simulink subsystem "Heater_Control"  (R2024b)
settings: Solver=VariableStepAuto  StartTime=0.0  StopTime=10.0  RelTol=1e-3
libraries: slident x1
settings Model: DataDictionary=Humidifier_Interface.sldd  EnableAccessToBaseWorkspace=off  Creator=ppatel  LastModifiedBy=ppatel

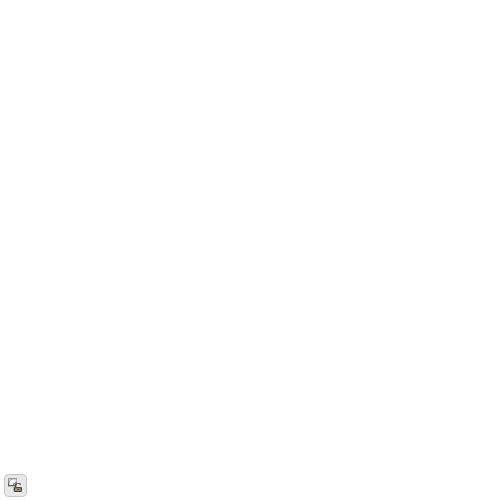
[thumbnail: Simulink's stored preview of the top-level diagram]
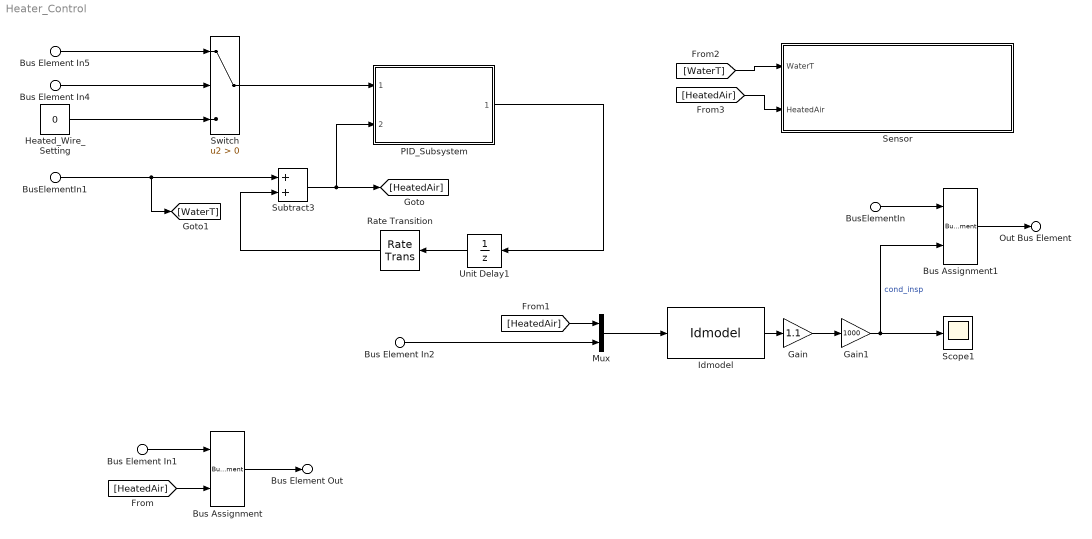
== system Heater_Control ==
  Bus Element In1 : Inport  PortName=HeaterT
  BusElementIn1 : Inport  PortName=HeaterT  Element=Water_T
  BusElementIn : Inport  Port=2  PortName=HeaterH
  Bus Element In2 : Inport  Port=2  PortName=HeaterH  Element=Humidifier_H
  Bus Element In4 : Inport  Port=3  PortName=auto_cnt
  Bus Element In5 : Inport  Port=4  PortName=heater  Element=Heater
  Bus Assignment : BusAssignment  AssignedSignals=heatedWire_T
  Bus Assignment1 : BusAssignment  AssignedSignals=CondLvl
  Gain : Gain  Gain=1.1
  Gain1 : Gain  Gain=1000
  Heated_Wire_Setting : Constant  Value=0
  Idmodel : slident/Models/Idmodel  sys=mp_heatedwire  IC=0  noi=on  seed=[]
  Mux : Mux  Inputs=2
  PID_Subsystem : Subsystem  ReferencedSubsystem=PIDSubsystem
      settings: PermitHierarchicalResolution=None
  Rate Transition : RateTransition
  Scope1 : Scope
  Sensor : Subsystem
  Subtract3 : Sum
  Switch : Switch  Criteria=u2 > Threshold  SaturateOnIntegerOverflow=off  InputSameDT=off
  Unit Delay1 : UnitDelay  SampleTime=-1  HasFrameUpgradeWarning=on
  Bus Element Out : Outport  PortName=wireT
  Out Bus Element : Outport  Port=2  PortName=heaterH
  wires:
  BusElementIn1/1 -> Subtract3/1, [WaterT]
  [HeatedAir] -> Sensor/2(HeatedAir)
  Bus Assignment/1 -> Bus Element Out/1
  Unit Delay1/1 -> Rate Transition/1
  Gain/1 -> Gain1/1
  Heated_Wire_Setting/1 -> Switch/3
  Mux/1 -> Idmodel/1
  [HeatedAir] -> Mux/1
  [HeatedAir] -> Bus Assignment/2
  Gain1/1 -> Scope1/1, Bus Assignment1/2  "cond_insp"
  Bus Element In2/1 -> Mux/2
  Switch/1 -> PID_Subsystem/1
  Bus Element In5/1 -> Switch/1
  Bus Element In4/1 -> Switch/2
  PID_Subsystem/1 -> Unit Delay1/1
  Bus Assignment1/1 -> Out Bus Element/1
  BusElementIn/1 -> Bus Assignment1/1
  Idmodel/1 -> Gain/1
  Bus Element In1/1 -> Bus Assignment/1
  [WaterT] -> Sensor/1(WaterT)
  Subtract3/1 -> [HeatedAir], PID_Subsystem/2
  Rate Transition/1 -> Subtract3/2

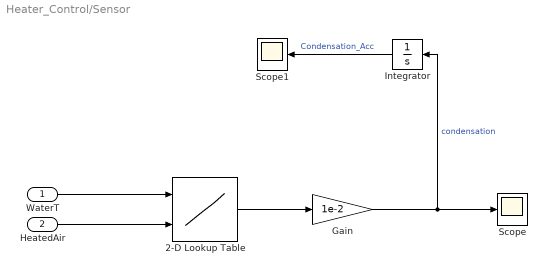
== system Heater_Control/Sensor ==
  WaterT : Inport
  HeatedAir : Inport  Port=2
  2-D Lookup Table : Lookup_n-D  BreakpointsForDimension1=[20 40 45]  BreakpointsForDimension2=[30;37]  Table=[1.75 2.5;2.2 3.1;2.5 3.5]  InternalRulePriority=Speed  RndMeth=Simplest
      settings: InputPortMap=u0,u1
  Gain : Gain  Gain=1e-2
  Integrator : Integrator
  Scope : Scope
  Scope1 : Scope
  wires:
  WaterT/1 -> 2-D Lookup Table/1
  HeatedAir/1 -> 2-D Lookup Table/2
  Gain/1 -> Scope/1, Integrator/1  "condensation"
  Integrator/1 -> Scope1/1  "Condensation_Acc"
  2-D Lookup Table/1 -> Gain/1
